simulink library "IOBlock_Library_TTC580"  (R2021a)
settings: Solver=ode45  StartTime=0.0  StopTime=10.0  RelTol=1e-3
PreLoadFcn:
  | addpath(genpath(fileparts(which('IOBlock_Library_TTC580'))));
  | %addpath(genpath(fileparts(which('IOBlock_Library_TTC580.mdl'))))
  | try
  | addpath(genpath([fileparts(which('IOBlock_Library_TTC580')),'\..\DBC_Importer']));
  | addpath(genpath([fileparts(which('IOBlock_Library_TTC580')),'\..\EEPROM_Importer']));
  | addpath(genpath([fileparts(which('IOBlock_Library_TTC580')),'\..\UserDoc']));
  | catch
  | warning('IOBlock_Library_TTC580: add path to DBC_Importer and EEPROM_Importer manually');
  | end
  | try
  | if exist('..\CustomPackage\scripts\OpenAllPackages.m','file')
  |      run('..\CustomPackage\scripts\OpenAllPackages.m'); %always available, ggf. empty
  | end
  | catch
  | warning('A problem occurred opening automatically the CustomPackage. Please open libraries manually');
  | end
  | try
  | set_param(0,'EditorSmartEditingHotParam','off');
  | catch
  | warning('Simlink preferences for ''Edit key parameter when adding new blocks'' needs to be unchecked manually');
  | end
undefined symbols (not defined in the file or in its folder): ADC_Absolute_10V, ADC_Absolute_32V, ADC_Absolute_5V, ADC_BoardTemp, ADC_ChannelInit, ADC_Current, ADC_Get, ADC_K15_, ADC_Ratiometric_10V, ADC_Ratiometric_5V, ADC_Resistive, ADC_SensorSupply, ADC_UBAT, bit_packing, bit_unpacking, CAN_ConfigMsg, compare2error, compare2FET_PROT_REENABLE, crc32_calc_intern, CRC32_EEPROM_Read, CRC32_EEPROM_Write, DIAG_EnterSafestate, DIAG_Status, DIAG_Status_internal, EEPROM_Mirror, EEPROM_Read, EEPROM_Read_OffsetIn, EEPROM_Read_Raw, EEPROM_Write, EEPROM_Write_OffsetIn, EEPROM_Write_Raw, EnterSafestate, FPU_Handler, Get_DI, Get_DI_VarThreshold, Get_K15_, Get_Pulse_Freq_Curr, Get_Pulse_Freq_Volt, Get_WakeUp, GetDateAndTime, IO_ADC_ResetProtection, IO_Blk_Lib_TTC500, IO_CAN_ReadMsg, IO_CAN_WriteMsg, IO_DI_Get, IO_DI_Init, IO_DI_Init_Var, IO_DO_GetCur, IO_DO_GetVoltage, IO_DO_Init, IO_DO_ResetProtection, IO_DO_Set, IO_Driver_GetSerialNumber, IO_Driver_GetVersionOfDriver, IO_Driver_GetVersionOfFPGA, IO_EEPROM_GetStatus, IO_EEPROM_Init, IO_EEPROM_Read_raw, IO_EEPROM_Write, IO_EEPROM_Write_OffsetIn ... (+73)
libraries: simulink x43
(part 11 of 18)

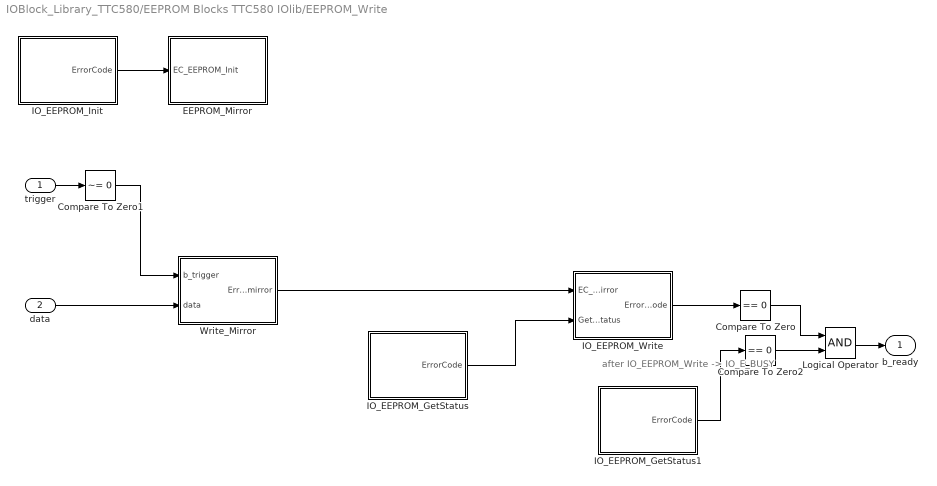
== system IOBlock_Library_TTC580/EEPROM Blocks TTC580 IOlib/EEPROM_Write ==
  note: after IO_EEPROM_Write -> IO_E_BUSY
  trigger : Inport
  data : Inport  Port=2  OutDataTypeStr=EEPROM_type
  Compare To Zero : simulink/Logic and Bit Operations/Compare To Zero  relop===  OutDataTypeStr=boolean  ZeroCross=off
  Compare To Zero1 : simulink/Logic and Bit Operations/Compare To Zero  relop=~=  OutDataTypeStr=boolean  ZeroCross=off
  Compare To Zero2 : simulink/Logic and Bit Operations/Compare To Zero  relop===  OutDataTypeStr=boolean  ZeroCross=off
  EEPROM_Mirror : Subsystem  LoadFcn=|  mask(EEPROM_Mirror_Code){SampleTime=-1, ttlib=IO_Blk_Lib_TTC500, ttDescription=EEPROM_Mirror, tt_iolib_version=0.21, offset=0, length=65536}
      | try
      | %
      | %Upgrade Information - standard BEGIN
      | new_color = 'blue';
      | new_ver = '0.21';
      | act_ver = get_param(gcb,'tt_iolib_version');
      | if not(strcmp(act_ver,new_ver))
      |     disp(['Upgrade block: ',gcb,char(10),'       Version: ',act_ver,' -> ',new_ver]);
      |     %switch - case for specific upgrade information e.g. additional parameter required 
      |     %Change appearance and version information
      |     set_param(gcb,'ForegroundColor',new_color);
      |     set_param(gcb,'tt_iolib_version',new_ver);
      | end
      | %Upgrade Information - standard END
      | catch
      | %Standard catch section BEGIN 
      | disp(' ');
      | disp('------------------------------------------------------------');
      | disp('An error occurred in a callback of the TTC580-BlockLib.');
      | disp(['Please check the parameters in the mask of ',gcb]);
      | disp('If you do not encounter any violations, then please '); 
      | disp('copy the following lines and report this to support@ttcontrol.com ');
      | disp('<< begin of error message dump >>');
      | disp(['Version of TTC580-BlockLib: ', get_param(gcb,'tt_iolib_version')]);
      | disp(get_param(gcb,'ttDescription'));
      | disp(gcb);
      | x=lasterror;disp(x.message);
      | disp(get_param(gcb,'MaskValues'));
      | disp(version);
      | disp(computer);
      | disp('<< end of error message dump >>');
      | disp('------------------------------------------------------------');
      | disp(' ');
      | %Standard catch section END
      | end
      mask help:
      | Read all data from the EEPROM and mirror this onto RAM.
      | The ErrorCode of IO_EEPROM_Init - block must be connected to the input of EEPROM_Mirror.
      | After calling EEPROM_Mirror the global variable EEPROM_mirror is filled and
      | the global variable ErrorCode_EEPROM_mirror contains the returns of IO_EEPROM_Init() and IO_EEPROM_Read().
      mask init:
      | %
      settings: CopyFcn=%deleted
      mask Help: web(which('IO_EEPROM.h'))
      mask Callback offset: %
      mask Callback length: %
  IO_EEPROM_GetStatus : Subsystem  LoadFcn=|  mask(IO_EEPROM_GetStatus_Code){SampleTime=-1, ttlib=IO_Blk_Lib_TTC500, ttDescription=IO_EEPROM_GetStatus, tt_iolib_version=0.19}
      | try
      | %
      | %Upgrade Information - standard BEGIN
      | new_color = 'blue';
      | new_ver = '0.19';
      | act_ver = get_param(gcb,'tt_iolib_version');
      | if not(strcmp(act_ver,new_ver))
      |     disp(['Upgrade block: ',gcb,char(10),'       Version: ',act_ver,' -> ',new_ver]);
      |     %switch - case for specific upgrade information e.g. additional parameter required 
      |     %Change appearance and version information
      |     set_param(gcb,'ForegroundColor',new_color);
      |     set_param(gcb,'tt_iolib_version',new_ver);
      | end
      | %Upgrade Information - standard END
      | catch
      | %Standard catch section BEGIN 
      | disp(' ');
      | disp('------------------------------------------------------------');
      | disp('An error occurred in a callback of the TTC580-BlockLib.');
      | disp(['Please check the parameters in the mask of ',gcb]);
      | disp('If you do not encounter any violations, then please '); 
      | disp('copy the following lines and report this to support@ttcontrol.com ');
      | disp('<< begin of error message dump >>');
      | disp(['Version of TTC580-BlockLib: ', get_param(gcb,'tt_iolib_version')]);
      | disp(get_param(gcb,'ttDescription'));
      | disp(gcb);
      | x=lasterror;disp(x.message);
      | disp(get_param(gcb,'MaskValues'));
      | disp(version);
      | disp(computer);
      | disp('<< end of error message dump >>');
      | disp('------------------------------------------------------------');
      | disp(' ');
      | %Standard catch section END
      | end
      mask help: Returns the status of the EEPROM driver.
      mask init:
      | %
      settings: CopyFcn=%deleted
      mask Help: web(which('IO_EEPROM.h'))
  IO_EEPROM_GetStatus1 : Subsystem  LoadFcn=|  mask(IO_EEPROM_GetStatus_Code){SampleTime=-1, ttlib=IO_Blk_Lib_TTC500, ttDescription=IO_EEPROM_GetStatus, tt_iolib_version=0.19}
      | try
      | %
      | %Upgrade Information - standard BEGIN
      | new_color = 'blue';
      | new_ver = '0.19';
      | act_ver = get_param(gcb,'tt_iolib_version');
      | if not(strcmp(act_ver,new_ver))
      |     disp(['Upgrade block: ',gcb,char(10),'       Version: ',act_ver,' -> ',new_ver]);
      |     %switch - case for specific upgrade information e.g. additional parameter required 
      |     %Change appearance and version information
      |     set_param(gcb,'ForegroundColor',new_color);
      |     set_param(gcb,'tt_iolib_version',new_ver);
      | end
      | %Upgrade Information - standard END
      | catch
      | %Standard catch section BEGIN 
      | disp(' ');
      | disp('------------------------------------------------------------');
      | disp('An error occurred in a callback of the TTC580-BlockLib.');
      | disp('Please copy the following lines and report this to support@tttech.com ');
      | disp('<< begin of error message dump >>');
      | disp(['Version of TTC580-BlockLib: ', get_param(gcb,'tt_iolib_version')]);
      | disp(get_param(gcb,'ttDescription'));
      | disp(gcb);
      | x=lasterror;disp(x.message);
      | disp(get_param(gcb,'MaskValues'));
      | disp(version);
      | disp(computer);
      | disp('<< end of error message dump >>');
      | disp('------------------------------------------------------------');
      | disp(' ');
      | %Standard catch section END
      | end
      mask help: Returns the status of the EEPROM driver.
      mask init:
      | %
      settings: CopyFcn=%deleted
      mask Help: web(which('IO_EEPROM.h'))
  IO_EEPROM_Init : Subsystem  LoadFcn=|  mask(IO_EEPROM_Init_Code){SampleTime=-1, ttlib=IO_Blk_Lib_TTC500, ttDescription=IO_EEPROM_Init, tt_iolib_version=0.19}
      | try
      | %
      | %Upgrade Information - standard BEGIN
      | new_color = 'blue';
      | new_ver = '0.19';
      | act_ver = get_param(gcb,'tt_iolib_version');
      | if not(strcmp(act_ver,new_ver))
      |     disp(['Upgrade block: ',gcb,char(10),'       Version: ',act_ver,' -> ',new_ver]);
      |     %switch - case for specific upgrade information e.g. additional parameter required 
      |     %Change appearance and version information
      |     set_param(gcb,'ForegroundColor',new_color);
      |     set_param(gcb,'tt_iolib_version',new_ver);
      | end
      | %Upgrade Information - standard END
      | catch
      | %Standard catch section BEGIN 
      | disp(' ');
      | disp('------------------------------------------------------------');
      | disp('An error occurred in a callback of the TTC580-BlockLib.');
      | disp(['Please check the parameters in the mask of ',gcb]);
      | disp('If you do not encounter any violations, then please '); 
      | disp('copy the following lines and report this to support@ttcontrol.com ');
      | disp('<< begin of error message dump >>');
      | disp(['Version of TTC580-BlockLib: ', get_param(gcb,'tt_iolib_version')]);
      | disp(get_param(gcb,'ttDescription'));
      | disp(gcb);
      | x=lasterror;disp(x.message);
      | disp(get_param(gcb,'MaskValues'));
      | disp(version);
      | disp(computer);
      | disp('<< end of error message dump >>');
      | disp('------------------------------------------------------------');
      | disp(' ');
      | %Standard catch section END
      | end
      mask help: Initialization of the EEPROM driver.
      mask init:
      | %
      settings: CopyFcn=%deleted
      mask Help: web(which('IO_EEPROM.h'))
  IO_EEPROM_Write : Subsystem  LoadFcn=|  mask(IO_EEPROM_Write_Code){SampleTime=-1, ttlib=IO_Blk_Lib_TTC500, ttDescription=IO_EEPROM_Write, tt_iolib_version=0.19, offset=offset, length=length}
      | try
      | %
      | %Upgrade Information - standard BEGIN
      | new_color = 'blue';
      | new_ver = '0.19';
      | act_ver = get_param(gcb,'tt_iolib_version');
      | if not(strcmp(act_ver,new_ver))
      |     disp(['Upgrade block: ',gcb,char(10),'       Version: ',act_ver,' -> ',new_ver]);
      |     %switch - case for specific upgrade information e.g. additional parameter required 
      |     %Change appearance and version information
      |     set_param(gcb,'ForegroundColor',new_color);
      |     set_param(gcb,'tt_iolib_version',new_ver);
      | end
      | %Upgrade Information - standard END
      | catch
      | %Standard catch section BEGIN 
      | disp(' ');
      | disp('------------------------------------------------------------');
      | disp('An error occurred in a callback of the TTC580-BlockLib.');
      | disp(['Please check the parameters in the mask of ',gcb]);
      | disp('If you do not encounter any violations, then please '); 
      | disp('copy the following lines and report this to support@ttcontrol.com ');
      | disp('<< begin of error message dump >>');
      | disp(['Version of TTC580-BlockLib: ', get_param(gcb,'tt_iolib_version')]);
      | disp(get_param(gcb,'ttDescription'));
      | disp(gcb);
      | x=lasterror;disp(x.message);
      | disp(get_param(gcb,'MaskValues'));
      | disp(version);
      | disp(computer);
      | disp('<< end of error message dump >>');
      | disp('------------------------------------------------------------');
      | disp(' ');
      | %Standard catch section END
      | end
      mask help:
      | Copy data from EEPROM_mirror[] to physical EEPROM. Copy activity is triggered by the edge of the input "EC_Write_Mirror" from IO_E_BUSY to IO_E_OK.
      | The output "ErrorCode" is IO_E_BUSY as long as writing to EEPROM is pending. During the activities are performed writing to the physical EEPROM, "ErrorCode" corresponds to the output of the C-driver IO_EEPROM_Write().
      mask init:
      | %
      settings: CopyFcn=%deleted
      mask Help: web(which('IO_EEPROM.h'))
      mask Callback offset: %
      mask Callback length: %
  Logical Operator : Logic  AllPortsSameDT=off  OutDataTypeStr=boolean
  Write_Mirror : Subsystem  LoadFcn=|  mask(Write_Mirror_Code){SampleTime=-1, ttlib=IO_Blk_Lib_TTC500, ttDescription=Write_Mirror, tt_iolib_version=0.19, offset=offset, length=length}
      | try
      | %
      | %Upgrade Information - standard BEGIN
      | new_color = 'blue';
      | new_ver = '0.19';
      | act_ver = get_param(gcb,'tt_iolib_version');
      | if not(strcmp(act_ver,new_ver))
      |     disp(['Upgrade block: ',gcb,char(10),'       Version: ',act_ver,' -> ',new_ver]);
      |     %switch - case for specific upgrade information e.g. additional parameter required 
      |     %Change appearance and version information
      |     set_param(gcb,'ForegroundColor',new_color);
      |     set_param(gcb,'tt_iolib_version',new_ver);
      | end
      | %Upgrade Information - standard END
      | catch
      | %Standard catch section BEGIN 
      | disp(' ');
      | disp('------------------------------------------------------------');
      | disp('An error occurred in a callback of the TTC580-BlockLib.');
      | disp(['Please check the parameters in the mask of ',gcb]);
      | disp('If you do not encounter any violations, then please '); 
      | disp('copy the following lines and report this to support@ttcontrol.com ');
      | disp('<< begin of error message dump >>');
      | disp(['Version of TTC580-BlockLib: ', get_param(gcb,'tt_iolib_version')]);
      | disp(get_param(gcb,'ttDescription'));
      | disp(gcb);
      | x=lasterror;disp(x.message);
      | disp(get_param(gcb,'MaskValues'));
      | disp(version);
      | disp(computer);
      | disp('<< end of error message dump >>');
      | disp('------------------------------------------------------------');
      | disp(' ');
      | %Standard catch section END
      | end
      mask help:
      | Write data to the mirror of the EEPROM. ErrorCode is set to IO_E_BUSY for one cycle of writing into EEPROM_mirror[].
      | In case the given data section exceeds given EEPROM boundaries, IO_E_EEPROM_RANGE ErrorCode is returned.
      mask init:
      | %
      settings: CopyFcn=%deleted
      mask Help: web(which('~.h'))
      mask Callback offset: %
      mask Callback length: %
  b_ready : Outport  VectorParamsAs1DForOutWhenUnconnected=off
  wires:
  IO_EEPROM_Write/1(ErrorCode) -> Compare To Zero/1
  trigger/1 -> Compare To Zero1/1
  data/1 -> Write_Mirror/2(data)
  IO_EEPROM_Init/1(ErrorCode) -> EEPROM_Mirror/1(EC_EEPROM_Init)
  Write_Mirror/1(ErrorCode_EEPROM_mirror) -> IO_EEPROM_Write/1(EC_Write_Mirror)
  IO_EEPROM_GetStatus/1(ErrorCode) -> IO_EEPROM_Write/2(GetStatus)
  Compare To Zero1/1 -> Write_Mirror/1(b_trigger)
  IO_EEPROM_GetStatus1/1(ErrorCode) -> Compare To Zero2/1
  Compare To Zero2/1 -> Logical Operator/2
  Logical Operator/1 -> b_ready/1
  Compare To Zero/1 -> Logical Operator/1

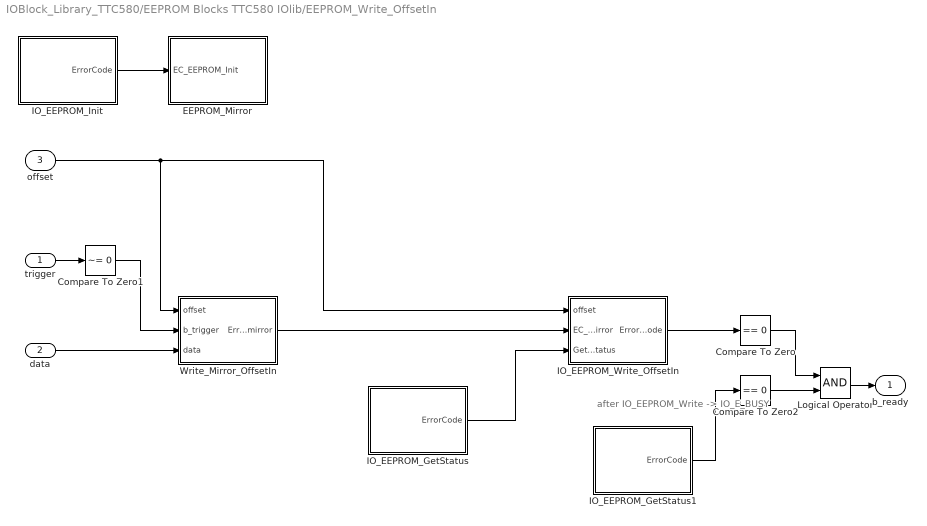
== system IOBlock_Library_TTC580/EEPROM Blocks TTC580 IOlib/EEPROM_Write_OffsetIn ==
  note: after IO_EEPROM_Write -> IO_E_BUSY
  trigger : Inport
  data : Inport  Port=2  OutDataTypeStr=EEPROM_type
  offset : Inport  Port=3  OutDataTypeStr=uint16  PortDimensions=1
  Compare To Zero : simulink/Logic and Bit Operations/Compare To Zero  relop===  OutDataTypeStr=boolean  ZeroCross=off
  Compare To Zero1 : simulink/Logic and Bit Operations/Compare To Zero  relop=~=  OutDataTypeStr=boolean  ZeroCross=off
  Compare To Zero2 : simulink/Logic and Bit Operations/Compare To Zero  relop===  OutDataTypeStr=boolean  ZeroCross=off
  EEPROM_Mirror : Subsystem  LoadFcn=|  mask(EEPROM_Mirror_Code){SampleTime=-1, ttlib=IO_Blk_Lib_TTC500, ttDescription=EEPROM_Mirror, tt_iolib_version=0.21, offset=0, length=65536}
      | try
      | %
      | %Upgrade Information - standard BEGIN
      | new_color = 'blue';
      | new_ver = '0.21';
      | act_ver = get_param(gcb,'tt_iolib_version');
      | if not(strcmp(act_ver,new_ver))
      |     disp(['Upgrade block: ',gcb,char(10),'       Version: ',act_ver,' -> ',new_ver]);
      |     %switch - case for specific upgrade information e.g. additional parameter required 
      |     %Change appearance and version information
      |     set_param(gcb,'ForegroundColor',new_color);
      |     set_param(gcb,'tt_iolib_version',new_ver);
      | end
      | %Upgrade Information - standard END
      | catch
      | %Standard catch section BEGIN 
      | disp(' ');
      | disp('------------------------------------------------------------');
      | disp('An error occurred in a callback of the TTC580-BlockLib.');
      | disp(['Please check the parameters in the mask of ',gcb]);
      | disp('If you do not encounter any violations, then please '); 
      | disp('copy the following lines and report this to support@ttcontrol.com ');
      | disp('<< begin of error message dump >>');
      | disp(['Version of TTC580-BlockLib: ', get_param(gcb,'tt_iolib_version')]);
      | disp(get_param(gcb,'ttDescription'));
      | disp(gcb);
      | x=lasterror;disp(x.message);
      | disp(get_param(gcb,'MaskValues'));
      | disp(version);
      | disp(computer);
      | disp('<< end of error message dump >>');
      | disp('------------------------------------------------------------');
      | disp(' ');
      | %Standard catch section END
      | end
      mask help:
      | Read all data from the EEPROM and mirror this onto RAM.
      | The ErrorCode of IO_EEPROM_Init - block must be connected to the input of EEPROM_Mirror.
      | After calling EEPROM_Mirror the global variable EEPROM_mirror is filled and
      | the global variable ErrorCode_EEPROM_mirror contains the returns of IO_EEPROM_Init() and IO_EEPROM_Read().
      mask init:
      | %
      settings: CopyFcn=%deleted
      mask Help: web(which('IO_EEPROM.h'))
      mask Callback offset: %
      mask Callback length: %
  IO_EEPROM_GetStatus : Subsystem  LoadFcn=|  mask(IO_EEPROM_GetStatus_Code){SampleTime=-1, ttlib=IO_Blk_Lib_TTC500, ttDescription=IO_EEPROM_GetStatus, tt_iolib_version=0.19}
      | try
      | %
      | %Upgrade Information - standard BEGIN
      | new_color = 'blue';
      | new_ver = '0.19';
      | act_ver = get_param(gcb,'tt_iolib_version');
      | if not(strcmp(act_ver,new_ver))
      |     disp(['Upgrade block: ',gcb,char(10),'       Version: ',act_ver,' -> ',new_ver]);
      |     %switch - case for specific upgrade information e.g. additional parameter required 
      |     %Change appearance and version information
      |     set_param(gcb,'ForegroundColor',new_color);
      |     set_param(gcb,'tt_iolib_version',new_ver);
      | end
      | %Upgrade Information - standard END
      | catch
      | %Standard catch section BEGIN 
      | disp(' ');
      | disp('------------------------------------------------------------');
      | disp('An error occurred in a callback of the TTC580-BlockLib.');
      | disp(['Please check the parameters in the mask of ',gcb]);
      | disp('If you do not encounter any violations, then please '); 
      | disp('copy the following lines and report this to support@ttcontrol.com ');
      | disp('<< begin of error message dump >>');
      | disp(['Version of TTC580-BlockLib: ', get_param(gcb,'tt_iolib_version')]);
      | disp(get_param(gcb,'ttDescription'));
      | disp(gcb);
      | x=lasterror;disp(x.message);
      | disp(get_param(gcb,'MaskValues'));
      | disp(version);
      | disp(computer);
      | disp('<< end of error message dump >>');
      | disp('------------------------------------------------------------');
      | disp(' ');
      | %Standard catch section END
      | end
      mask help: Returns the status of the EEPROM driver.
      mask init:
      | %
      settings: CopyFcn=%deleted
      mask Help: web(which('IO_EEPROM.h'))
  IO_EEPROM_GetStatus1 : Subsystem  LoadFcn=|  mask(IO_EEPROM_GetStatus_Code){SampleTime=-1, ttlib=IO_Blk_Lib_TTC500, ttDescription=IO_EEPROM_GetStatus, tt_iolib_version=0.19}
      | try
      | %
      | %Upgrade Information - standard BEGIN
      | new_color = 'blue';
      | new_ver = '0.19';
      | act_ver = get_param(gcb,'tt_iolib_version');
      | if not(strcmp(act_ver,new_ver))
      |     disp(['Upgrade block: ',gcb,char(10),'       Version: ',act_ver,' -> ',new_ver]);
      |     %switch - case for specific upgrade information e.g. additional parameter required 
      |     %Change appearance and version information
      |     set_param(gcb,'ForegroundColor',new_color);
      |     set_param(gcb,'tt_iolib_version',new_ver);
      | end
      | %Upgrade Information - standard END
      | catch
      | %Standard catch section BEGIN 
      | disp(' ');
      | disp('------------------------------------------------------------');
      | disp('An error occurred in a callback of the TTC580-BlockLib.');
      | disp('Please copy the following lines and report this to support@tttech.com ');
      | disp('<< begin of error message dump >>');
      | disp(['Version of TTC580-BlockLib: ', get_param(gcb,'tt_iolib_version')]);
      | disp(get_param(gcb,'ttDescription'));
      | disp(gcb);
      | x=lasterror;disp(x.message);
      | disp(get_param(gcb,'MaskValues'));
      | disp(version);
      | disp(computer);
      | disp('<< end of error message dump >>');
      | disp('------------------------------------------------------------');
      | disp(' ');
      | %Standard catch section END
      | end
      mask help: Returns the status of the EEPROM driver.
      mask init:
      | %
      settings: CopyFcn=%deleted
      mask Help: web(which('IO_EEPROM.h'))
  IO_EEPROM_Init : Subsystem  LoadFcn=|  mask(IO_EEPROM_Init_Code){SampleTime=-1, ttlib=IO_Blk_Lib_TTC500, ttDescription=IO_EEPROM_Init, tt_iolib_version=0.19}
      | try
      | %
      | %Upgrade Information - standard BEGIN
      | new_color = 'blue';
      | new_ver = '0.19';
      | act_ver = get_param(gcb,'tt_iolib_version');
      | if not(strcmp(act_ver,new_ver))
      |     disp(['Upgrade block: ',gcb,char(10),'       Version: ',act_ver,' -> ',new_ver]);
      |     %switch - case for specific upgrade information e.g. additional parameter required 
      |     %Change appearance and version information
      |     set_param(gcb,'ForegroundColor',new_color);
      |     set_param(gcb,'tt_iolib_version',new_ver);
      | end
      | %Upgrade Information - standard END
      | catch
      | %Standard catch section BEGIN 
      | disp(' ');
      | disp('------------------------------------------------------------');
      | disp('An error occurred in a callback of the TTC580-BlockLib.');
      | disp(['Please check the parameters in the mask of ',gcb]);
      | disp('If you do not encounter any violations, then please '); 
      | disp('copy the following lines and report this to support@ttcontrol.com ');
      | disp('<< begin of error message dump >>');
      | disp(['Version of TTC580-BlockLib: ', get_param(gcb,'tt_iolib_version')]);
      | disp(get_param(gcb,'ttDescription'));
      | disp(gcb);
      | x=lasterror;disp(x.message);
      | disp(get_param(gcb,'MaskValues'));
      | disp(version);
      | disp(computer);
      | disp('<< end of error message dump >>');
      | disp('------------------------------------------------------------');
      | disp(' ');
      | %Standard catch section END
      | end
      mask help: Initialization of the EEPROM driver.
      mask init:
      | %
      settings: CopyFcn=%deleted
      mask Help: web(which('IO_EEPROM.h'))
  IO_EEPROM_Write_OffsetIn : Subsystem  LoadFcn=|  mask(IO_EEPROM_Write_OffsetIn_Code){SampleTime=-1, ttlib=IO_Blk_Lib_TTC500, ttDescription=IO_EEPROM_Write_OffsetIn, tt_iolib_version=0.23, length=length}
      | try
      | %
      | %Upgrade Information - standard BEGIN
      | new_color = 'blue';
      | new_ver = '0.23';
      | act_ver = get_param(gcb,'tt_iolib_version');
      | if not(strcmp(act_ver,new_ver))
      |     disp(['Upgrade block: ',gcb,char(10),'       Version: ',act_ver,' -> ',new_ver]);
      |     %switch - case for specific upgrade information e.g. additional parameter required 
      |     %Change appearance and version information
      |     set_param(gcb,'ForegroundColor',new_color);
      |     set_param(gcb,'tt_iolib_version',new_ver);
      | end
      | %Upgrade Information - standard END
      | catch
      | %Standard catch section BEGIN 
      | disp(' ');
      | disp('------------------------------------------------------------');
      | disp('An error occurred in a callback of the TTC580-BlockLib.');
      | disp(['Please check the parameters in the mask of ',gcb]);
      | disp('If you do not encounter any violations, then please '); 
      | disp('copy the following lines and report this to support@ttcontrol.com ');
      | disp('<< begin of error message dump >>');
      | disp(['Version of TTC580-BlockLib: ', get_param(gcb,'tt_iolib_version')]);
      | disp(get_param(gcb,'ttDescription'));
      | disp(gcb);
      | x=lasterror;disp(x.message);
      | disp(get_param(gcb,'MaskValues'));
      | disp(version);
      | disp(computer);
      | disp('<< end of error message dump >>');
      | disp('------------------------------------------------------------');
      | disp(' ');
      | %Standard catch section END
      | end
      mask help:
      | Copy data from EEPROM_mirror[] to physical EEPROM. Copy activity is triggered by the edge of the input "EC_Write_Mirror" from IO_E_BUSY to IO_E_OK.
      | The output "ErrorCode" is IO_E_BUSY as long as writing to EEPROM is pending. During the activities are performed writing to the physical EEPROM,"ErrorCode" corresponds to the output of the C-driver IO_EEPROM_Write().
      mask init:
      | %
      settings: CopyFcn=%deleted
      mask Help: No further help available for this block
      mask Callback length: %
  Logical Operator : Logic  AllPortsSameDT=off  OutDataTypeStr=boolean
  Write_Mirror_OffsetIn : Subsystem  LoadFcn=|  mask(Write_Mirror_OffsetIn_Code){SampleTime=-1, ttlib=IO_Blk_Lib_TTC500, ttDescription=Write_Mirror_OffsetIn, tt_iolib_version=0.23, length=length}
      | try
      | %
      | %Upgrade Information - standard BEGIN
      | new_color = 'blue';
      | new_ver = '0.23';
      | act_ver = get_param(gcb,'tt_iolib_version');
      | if not(strcmp(act_ver,new_ver))
      |     disp(['Upgrade block: ',gcb,char(10),'       Version: ',act_ver,' -> ',new_ver]);
      |     %switch - case for specific upgrade information e.g. additional parameter required 
      |     %Change appearance and version information
      |     set_param(gcb,'ForegroundColor',new_color);
      |     set_param(gcb,'tt_iolib_version',new_ver);
      | end
      | %Upgrade Information - standard END
      | catch
      | %Standard catch section BEGIN 
      | disp(' ');
      | disp('------------------------------------------------------------');
      | disp('An error occurred in a callback of the TTC580-BlockLib.');
      | disp(['Please check the parameters in the mask of ',gcb]);
      | disp('If you do not encounter any violations, then please '); 
      | disp('copy the following lines and report this to support@ttcontrol.com ');
      | disp('<< begin of error message dump >>');
      | disp(['Version of TTC580-BlockLib: ', get_param(gcb,'tt_iolib_version')]);
      | disp(get_param(gcb,'ttDescription'));
      | disp(gcb);
      | x=lasterror;disp(x.message);
      | disp(get_param(gcb,'MaskValues'));
      | disp(version);
      | disp(computer);
      | disp('<< end of error message dump >>');
      | disp('------------------------------------------------------------');
      | disp(' ');
      | %Standard catch section END
      | end
      mask help:
      | Write data to the mirror of the EEPROM. ErrorCode is set to IO_E_BUSY for one cycle of writing into EEPROM_mirror[].
      | In case the given data section exceeds given EEPROM boundaries, IO_E_EEPROM_RANGE ErrorCode is returned.
      mask init:
      | %
      settings: CopyFcn=%deleted
      mask Help: No further help available for this block
      mask Callback length: %
  b_ready : Outport  VectorParamsAs1DForOutWhenUnconnected=off
  wires:
  IO_EEPROM_Write_OffsetIn/1(ErrorCode) -> Compare To Zero/1
  trigger/1 -> Compare To Zero1/1
  IO_EEPROM_Init/1(ErrorCode) -> EEPROM_Mirror/1(EC_EEPROM_Init)
  Write_Mirror_OffsetIn/1(ErrorCode_EEPROM_mirror) -> IO_EEPROM_Write_OffsetIn/2(EC_Write_Mirror)
  IO_EEPROM_GetStatus/1(ErrorCode) -> IO_EEPROM_Write_OffsetIn/3(GetStatus)
  Compare To Zero1/1 -> Write_Mirror_OffsetIn/2(b_trigger)
  data/1 -> Write_Mirror_OffsetIn/3(data)
  offset/1 -> IO_EEPROM_Write_OffsetIn/1(offset), Write_Mirror_OffsetIn/1(offset)
  IO_EEPROM_GetStatus1/1(ErrorCode) -> Compare To Zero2/1
  Compare To Zero/1 -> Logical Operator/1
  Compare To Zero2/1 -> Logical Operator/2
  Logical Operator/1 -> b_ready/1

== system IOBlock_Library_TTC580/EEPROM Blocks TTC580 IOlib/EEPROM_Write_Raw ==
  data : Inport  OutDataTypeStr=EEPROM_type
  IO_EEPROM_Init : Subsystem  LoadFcn=|  mask(IO_EEPROM_Init_Code){SampleTime=-1, ttlib=IO_Blk_Lib_TTC500, ttDescription=IO_EEPROM_Init, tt_iolib_version=0.24}
      | try
      | %
      | %Upgrade Information - standard BEGIN
      | new_color = 'blue';
      | new_ver = '0.24';
      | act_ver = get_param(gcb,'tt_iolib_version');
      | if not(strcmp(act_ver,new_ver))
      |     disp(['Upgrade block: ',gcb,char(10),'       Version: ',act_ver,' -> ',new_ver]);
      |     %switch - case for specific upgrade information e.g. additional parameter required 
      |     %Change appearance and version information
      |     set_param(gcb,'ForegroundColor',new_color);
      |     set_param(gcb,'tt_iolib_version',new_ver);
      | end
      | %Upgrade Information - standard END
      | catch
      | %Standard catch section BEGIN 
      | disp(' ');
      | disp('------------------------------------------------------------');
      | disp('An error occurred in a callback of the TTC580-BlockLib.');
      | disp(['Please check the parameters in the mask of ',gcb]);
      | disp('If you do not encounter any violations, then please '); 
      | disp('copy the following lines and report this to support@ttcontrol.com ');
      | disp('<< begin of error message dump >>');
      | disp(['Version of TTC580-BlockLib: ', get_param(gcb,'tt_iolib_version')]);
      | disp(get_param(gcb,'ttDescription'));
      | disp(gcb);
      | x=lasterror;disp(x.message);
      | disp(get_param(gcb,'MaskValues'));
      | disp(version);
      | disp(computer);
      | disp('<< end of error message dump >>');
      | disp('------------------------------------------------------------');
      | disp(' ');
      | %Standard catch section END
      | end
      mask help: Initialization of the EEPROM driver.
      mask init:
      | %
      settings: CopyFcn=%deleted
      mask Help: No further help available for this block
  IO_EEPROM_Write_raw : Subsystem  LoadFcn=|  mask(IO_EEPROM_Write_raw_Code){SampleTime=-1, ttlib=IO_Blk_Lib_TTC500, ttDescription=IO_EEPROM_Write_raw, tt_iolib_version=0.24, offset=offset, length=length}
      | try
      | %
      | %Upgrade Information - standard BEGIN
      | new_color = 'blue';
      | new_ver = '0.24';
      | act_ver = get_param(gcb,'tt_iolib_version');
      | if not(strcmp(act_ver,new_ver))
      |     disp(['Upgrade block: ',gcb,char(10),'       Version: ',act_ver,' -> ',new_ver]);
      |     %switch - case for specific upgrade information e.g. additional parameter required 
      |     %Change appearance and version information
      |     set_param(gcb,'ForegroundColor',new_color);
      |     set_param(gcb,'tt_iolib_version',new_ver);
      | end
      | %Upgrade Information - standard END
      | catch
      | %Standard catch section BEGIN 
      | disp(' ');
      | disp('------------------------------------------------------------');
      | disp('An error occurred in a callback of the TTC580-BlockLib.');
      | disp(['Please check the parameters in the mask of ',gcb]);
      | disp('If you do not encounter any violations, then please '); 
      | disp('copy the following lines and report this to support@ttcontrol.com ');
      | disp('<< begin of error message dump >>');
      | disp(['Version of TTC580-BlockLib: ', get_param(gcb,'tt_iolib_version')]);
      | disp(get_param(gcb,'ttDescription'));
      | disp(gcb);
      | x=lasterror;disp(x.message);
      | disp(get_param(gcb,'MaskValues'));
      | disp(version);
      | disp(computer);
      | disp('<< end of error message dump >>');
      | disp('------------------------------------------------------------');
      | disp(' ');
      | %Standard catch section END
      | end
      mask help: Write data to EEPROM
      mask init:
      | %
      settings: CopyFcn=%deleted
      mask Help: No further help available for this block
      mask Callback offset: %
      mask Callback length: %
  Terminator : Terminator
  ErrorCode : Outport  VectorParamsAs1DForOutWhenUnconnected=off
  wires:
  IO_EEPROM_Init/1(ErrorCode) -> Terminator/1
  IO_EEPROM_Write_raw/1(ErrorCode) -> ErrorCode/1
  data/1 -> IO_EEPROM_Write_raw/1(data)

== system IOBlock_Library_TTC580/EEPROM Blocks TTC580 IOlib/IO_EEPROM_GetStatus ==
  IO_EEPROM_GetStatus_s : S-Function  FunctionName=IO_EEPROM_GetStatus_s  Parameters=SampleTime  SFunctionDeploymentMode=off  EnableBusSupport=off
  ErrorCode : Outport  VectorParamsAs1DForOutWhenUnconnected=off
  wires:
  IO_EEPROM_GetStatus_s/1 -> ErrorCode/1

== system IOBlock_Library_TTC580/Examples/Example_ADC ==
  Ground : Ground
  Terminator : Terminator
  wires:
  Ground/1 -> Terminator/1

== system IOBlock_Library_TTC580/Examples/Example_CAN ==
  Ground : Ground
  Terminator : Terminator
  wires:
  Ground/1 -> Terminator/1

== system IOBlock_Library_TTC580/Examples/Example_CustomCode ==
  Ground : Ground
  Terminator : Terminator
  wires:
  Ground/1 -> Terminator/1

== system IOBlock_Library_TTC580/Examples/Example_DBCImporter ==
  Ground : Ground
  Terminator : Terminator
  wires:
  Ground/1 -> Terminator/1

== system IOBlock_Library_TTC580/Examples/Example_DI_DO ==
  Ground : Ground
  Terminator : Terminator
  wires:
  Ground/1 -> Terminator/1

== system IOBlock_Library_TTC580/Examples/Example_EEPROM ==
  Ground : Ground
  Terminator : Terminator
  wires:
  Ground/1 -> Terminator/1

== system IOBlock_Library_TTC580/Examples/Example_EEPROM1 ==
  Ground : Ground
  Terminator : Terminator
  wires:
  Ground/1 -> Terminator/1

== system IOBlock_Library_TTC580/Examples/Example_EEPROM2 ==
  Ground : Ground
  Terminator : Terminator
  wires:
  Ground/1 -> Terminator/1

== system IOBlock_Library_TTC580/Examples/Example_EEPROMImporter ==
  Ground : Ground
  Terminator : Terminator
  wires:
  Ground/1 -> Terminator/1

== system IOBlock_Library_TTC580/Examples/Example_FPUHandler ==
  Ground : Ground
  Terminator : Terminator
  wires:
  Ground/1 -> Terminator/1

== system IOBlock_Library_TTC580/Examples/Example_GetSerialNumber ==
  Ground : Ground
  Terminator : Terminator
  wires:
  Ground/1 -> Terminator/1

== system IOBlock_Library_TTC580/Examples/Example_LIN ==
  Ground : Ground
  Terminator : Terminator
  wires:
  Ground/1 -> Terminator/1

== system IOBlock_Library_TTC580/Examples/Example_ModelRef ==
  Ground : Ground
  Terminator : Terminator
  wires:
  Ground/1 -> Terminator/1

== system IOBlock_Library_TTC580/Examples/Example_PWD ==
  Ground : Ground
  Terminator : Terminator
  wires:
  Ground/1 -> Terminator/1

== system IOBlock_Library_TTC580/Examples/Example_PWM ==
  Ground : Ground
  Terminator : Terminator
  wires:
  Ground/1 -> Terminator/1

== system IOBlock_Library_TTC580/Examples/Example_Power ==
  Ground : Ground
  Terminator : Terminator
  wires:
  Ground/1 -> Terminator/1

== system IOBlock_Library_TTC580/Examples/Example_RTC ==
  Ground : Ground
  Terminator : Terminator
  wires:
  Ground/1 -> Terminator/1

== system IOBlock_Library_TTC580/Examples/Example_SensorSupply ==
  Ground : Ground
  Terminator : Terminator
  wires:
  Ground/1 -> Terminator/1

== system IOBlock_Library_TTC580/Examples/Example_UART ==
  Ground : Ground
  Terminator : Terminator
  wires:
  Ground/1 -> Terminator/1

== system IOBlock_Library_TTC580/Examples/Example_UART1 ==
  Ground : Ground
  Terminator : Terminator
  wires:
  Ground/1 -> Terminator/1

== system IOBlock_Library_TTC580/Examples/Example_VOUT_PVG ==
  Ground : Ground
  Terminator : Terminator
  wires:
  Ground/1 -> Terminator/1

== system IOBlock_Library_TTC580/Examples/Info ==
  Ground : Ground
  Terminator : Terminator
  wires:
  Ground/1 -> Terminator/1

== system IOBlock_Library_TTC580/LIN TTC580 IOlib/IO_LIN_GetStatus ==
  IO_LIN_GetStatus_s : S-Function  FunctionName=IO_LIN_GetStatus_s  Parameters=SampleTime  SFunctionDeploymentMode=off  EnableBusSupport=off
  ErrorCode : Outport  VectorParamsAs1DForOutWhenUnconnected=off
  wires:
  IO_LIN_GetStatus_s/1 -> ErrorCode/1

== system IOBlock_Library_TTC580/LIN TTC580 IOlib/IO_LIN_Init ==
  Constant : Constant  Value=LIN_baudrate  OutDataTypeStr=uint16
  Constant1 : Constant  Value=(LIN_checksum_type - 1) %popup entry - 1  OutDataTypeStr=uint8
  IO_LIN_Init : Subsystem  LoadFcn=|  mask(IO_LIN_Init_Code){SampleTime=-1, ttlib=IO_Blk_Lib_TTC500, ttDescription=IO_LIN_Init, tt_iolib_version=0.24}
      | try
      | %
      | %Upgrade Information - standard BEGIN
      | new_color = 'blue';
      | new_ver = '0.24';
      | act_ver = get_param(gcb,'tt_iolib_version');
      | if not(strcmp(act_ver,new_ver))
      |     disp(['Upgrade block: ',gcb,char(10),'       Version: ',act_ver,' -> ',new_ver]);
      |     %switch - case for specific upgrade information e.g. additional parameter required 
      |     %Change appearance and version information
      |     set_param(gcb,'ForegroundColor',new_color);
      |     set_param(gcb,'tt_iolib_version',new_ver);
      | end
      | %Upgrade Information - standard END
      | catch
      | %Standard catch section BEGIN 
      | disp(' ');
      | disp('------------------------------------------------------------');
      | disp('An error occurred in a callback of the TTC580-BlockLib.');
      | disp(['Please check the parameters in the mask of ',gcb]);
      | disp('If you do not encounter any violations, then please '); 
      | disp('copy the following lines and report this to support@ttcontrol.com ');
      | disp('<< begin of error message dump >>');
      | disp(['Version of TTC580-BlockLib: ', get_param(gcb,'tt_iolib_version')]);
      | disp(get_param(gcb,'ttDescription'));
      | disp(gcb);
      | x=lasterror;disp(x.message);
      | disp(get_param(gcb,'MaskValues'));
      | disp(version);
      | disp(computer);
      | disp('<< end of error message dump >>');
      | disp('------------------------------------------------------------');
      | disp(' ');
      | %Standard catch section END
      | end
      mask help: Initialization of the LIN communication driver.
      settings: CopyFcn=%deleted
      mask Help: No further help available for this block
  ErrorCode : Outport  VectorParamsAs1DForOutWhenUnconnected=off
  wires:
  Constant1/1 -> IO_LIN_Init/2(checksum_type)
  Constant/1 -> IO_LIN_Init/1(baudrate)
  IO_LIN_Init/1(ErrorCode) -> ErrorCode/1

== system IOBlock_Library_TTC580/LIN TTC580 IOlib/LIN_Read ==
  note: make sure that data
      | has exactly the width
      | of frame_length !
  b_reqst : Inport  OutDataTypeStr=boolean  PortDimensions=1
  Constant : Constant  Value=(LIN_id -1) %from popup: starts with 1  OutDataTypeStr=uint8
  Constant1 : Constant  Value=LIN_length  OutDataTypeStr=uint8
  LIN_Read_intern : Subsystem  LoadFcn=|  mask(LIN_Read_intern_Code){SampleTime=-1, ttlib=IO_Blk_Lib_TTC500, ttDescription=LIN_Read_intern, tt_iolib_version=0.24}
      | try
      | %
      | %Upgrade Information - standard BEGIN
      | new_color = 'blue';
      | new_ver = '0.24';
      | act_ver = get_param(gcb,'tt_iolib_version');
      | if not(strcmp(act_ver,new_ver))
      |     disp(['Upgrade block: ',gcb,char(10),'       Version: ',act_ver,' -> ',new_ver]);
      |     %switch - case for specific upgrade information e.g. additional parameter required 
      |     %Change appearance and version information
      |     set_param(gcb,'ForegroundColor',new_color);
      |     set_param(gcb,'tt_iolib_version',new_ver);
      | end
      | %Upgrade Information - standard END
      | catch
      | %Standard catch section BEGIN 
      | disp(' ');
      | disp('------------------------------------------------------------');
      | disp('An error occurred in a callback of the TTC580-BlockLib.');
      | disp(['Please check the parameters in the mask of ',gcb]);
      | disp('If you do not encounter any violations, then please '); 
      | disp('copy the following lines and report this to support@ttcontrol.com ');
      | disp('<< begin of error message dump >>');
      | disp(['Version of TTC580-BlockLib: ', get_param(gcb,'tt_iolib_version')]);
      | disp(get_param(gcb,'ttDescription'));
      | disp(gcb);
      | x=lasterror;disp(x.message);
      | disp(get_param(gcb,'MaskValues'));
      | disp(version);
      | disp(computer);
      | disp('<< end of error message dump >>');
      | disp('------------------------------------------------------------');
      | disp(' ');
      | %Standard catch section END
      | end
      mask help:
      | Reads a LIN frame with the given id and of the given length.
      | Width of output data always needs to be set to given length by the user.
      mask init:
      | %
      settings: CopyFcn=%deleted
      mask Help: No further help available for this block
  ErrorCode : Outport  VectorParamsAs1DForOutWhenUnconnected=off
  data : Outport  Port=2  OutDataTypeStr=uint8  PortDimensions=LIN_length  VectorParamsAs1DForOutWhenUnconnected=off
  wires:
  b_reqst/1 -> LIN_Read_intern/3(b_reqst)
  LIN_Read_intern/1(ErrorCode) -> ErrorCode/1
  LIN_Read_intern/2(frame_data) -> data/1
  Constant/1 -> LIN_Read_intern/1(frame_id)
  Constant1/1 -> LIN_Read_intern/2(frame_length)

== system IOBlock_Library_TTC580/LIN TTC580 IOlib/LIN_Write ==
  note: make sure that data
      | has exactly the width
      | of frame_length !
  b_send : Inport  OutDataTypeStr=boolean  PortDimensions=1
  data : Inport  Port=2  OutDataTypeStr=uint8  PortDimensions=LIN_length
  Constant : Constant  Value=(LIN_id -1) %from popup: starts with 1  OutDataTypeStr=uint8
  Constant1 : Constant  Value=LIN_length  OutDataTypeStr=uint8
  IO_LIN_Write : Subsystem  LoadFcn=|  mask(IO_LIN_Write_Code){SampleTime=-1, ttlib=IO_Blk_Lib_TTC500, ttDescription=IO_LIN_Write, tt_iolib_version=0.24}
      | try
      | %
      | %Upgrade Information - standard BEGIN
      | new_color = 'blue';
      | new_ver = '0.24';
      | act_ver = get_param(gcb,'tt_iolib_version');
      | if not(strcmp(act_ver,new_ver))
      |     disp(['Upgrade block: ',gcb,char(10),'       Version: ',act_ver,' -> ',new_ver]);
      |     %switch - case for specific upgrade information e.g. additional parameter required 
      |     %Change appearance and version information
      |     set_param(gcb,'ForegroundColor',new_color);
      |     set_param(gcb,'tt_iolib_version',new_ver);
      | end
      | %Upgrade Information - standard END
      | catch
      | %Standard catch section BEGIN 
      | disp(' ');
      | disp('------------------------------------------------------------');
      | disp('An error occurred in a callback of the TTC580-BlockLib.');
      | disp(['Please check the parameters in the mask of ',gcb]);
      | disp('If you do not encounter any violations, then please '); 
      | disp('copy the following lines and report this to support@ttcontrol.com ');
      | disp('<< begin of error message dump >>');
      | disp(['Version of TTC580-BlockLib: ', get_param(gcb,'tt_iolib_version')]);
      | disp(get_param(gcb,'ttDescription'));
      | disp(gcb);
      | x=lasterror;disp(x.message);
      | disp(get_param(gcb,'MaskValues'));
      | disp(version);
      | disp(computer);
      | disp('<< end of error message dump >>');
      | disp('------------------------------------------------------------');
      | disp(' ');
      | %Standard catch section END
      | end
      mask help:
      | Transmit a LIN frame with the given id and of the given length.
      | Width of input data always needs to be set to given length by the user.
      mask init:
      | %
      settings: CopyFcn=%deleted
      mask Help: No further help available for this block
  ErrorCode : Outport  VectorParamsAs1DForOutWhenUnconnected=off
  wires:
  Constant/1 -> IO_LIN_Write/1(frame_id)
  Constant1/1 -> IO_LIN_Write/2(frame_length)
  IO_LIN_Write/1(ErrorCode) -> ErrorCode/1
  data/1 -> IO_LIN_Write/3(frame_data)
  b_send/1 -> IO_LIN_Write/Enable
